simulink model "SF049A_LoaMgr"  (R2013b)
settings: Solver=FixedStepDiscrete  SolverMode=SingleTasking  StartTime=0.0  StopTime=1  FixedStep=0.002  RelTol=1e-3
undefined symbols (not defined in the file): CURRMEASLOAMTGTNMASK_CNT_U08, IVTRLOAMTGTNMASK_CNT_U08, LoaCtrldShtdwn, LoaCurrMeasIdptSigNrFlt, LoaHwTqIdptSigNrFlt, LoaImdtShtdwn, LoaIvtrIdptSigNrFlt, LOAMAXSLEW_ULSPERSEC_F32, LoaMgrCurrIvtrMtgtnRate, LoaMgrCurrIvtrMtgtnSca, LoaMgrCurrIvtrMtgtnScaZeroEna, LoaMgrCurrMeasIdptSig0Resp, LoaMgrCurrMeasIdptSig1Resp, LoaMgrCurrMeasIdptSig2Resp, LoaMgrCurrMeasIdptSigFltThd, LoaMgrCurrMeasMtgtnRate, LoaMgrCurrMeasMtgtnSca, LoaMgrCurrMeasMtgtnScaZeroEna, LoaMgrFadeOutStRate, LoaMgrHwTqIdptSig0NoTqLoaResp, LoaMgrHwTqIdptSig1NoTqLoaResp, LoaMgrHwTqIdptSig2Resp, LoaMgrHwTqIdptSig4Resp, LoaMgrHwTqIdptSigFltThd, LoaMgrHwTqLoaAvlResp, LoaMgrIvtrIdptSig0Resp, LoaMgrIvtrIdptSig1Resp, LoaMgrIvtrIdptSig2Resp, LoaMgrIvtrIdptSigFltThd, LoaMgrIvtrMtgtnRate, LoaMgrIvtrMtgtnSca, LoaMgrIvtrMtgtnScaZeroEna, LoaMgrLimdStRate, LoaMgrLimdStSca, LoaMgrMotAgAvlSnsrlsResp, LoaMgrMotAgIdptSig0NoSnsrlsResp, LoaMgrMotAgIdptSig1NoSnsrlsResp, LoaMgrMotAgIdptSig2Resp, LoaMgrMotAgIdptSig3Resp, LoaMgrMotAgIdptSigFltThd, LoaMgrMotAgMtgtnRate, LoaMgrMotAgMtgtnSca, LoaMgrMotAgMtgtnScaZeroEna, LoaMotAgIdptSigNrFlt, LOASCAONE_ULS_F32, LOASCAZERO_ULS_F32, LoaSt1, LOASTIMDTSHTDWN_CNT_U08, LOASTNORM_CNT_U08, LOASTSWMTGTN_CNT_U08, MAXCURRMEASIDPTSIGALLWD_CNT_U08, MAXHWTQIDPTSIGALLWD_CNT_U08, MAXIVTRIDPTSIGALLWD_CNT_U08, MAXMOTAGMECLIDPTSIGALLWD_CNT_U08, NODEBSTEP_CNT_U16, NtcSts1, SigQlfr1
libraries: simulink x30, NxtrMin x4, NxtrMax x4, NxtrLim x2
(part 6 of 7)

== system SF049A_LoaMgr/LoaMgr/LoaMgrPer1/Assign_Scale/SwMtgtn/OthersTrue ==
  note: Value Assignments
      |   0  neither enabled (shouldn't get here if this is true)
      |   1  MotCurrLoaMtgtnEn
      |   2  IvtrLoaMtgtnEn
      |   3  both enabled
  note: Set case 3 as the default.
  VltgModSrc : Inport  RequirementInfo={} %GIDa_e34c3d9f_9321_4084_85fd_c576df9628c2
  PrevVltgModSrc : Inport  RequirementInfo={} %GIDa_5c8ae546_718f_4248_8614_1d27d062207c  Port=2
  Action Port : ActionPort  ActionType=else
  CopyRight2 : Subsystem  Description=|  mask(Copyright Information){none=on}
      | Copyright info block.                                               
      |                                                                     
      | Place copyright information at the top of every subsystem in design.
      mask prompts: none "No parameters"
      mask help: Place copyright information at the top of every subsystem in design.
      mask Display:
      | NxtrConf = 'Nexteer Confidential';
      | 
      | sys = bdroot; %handle for the current model ("system")
      | first = get_param(sys,'Created');
      | first = first(end-3:end);  %year is last four digits
      | 
      | last = get_param(sys,'LastModifiedDate');
      | if isempty(last)
      |     last = datestr(now,'yyyy');
      | else
      |     last = last(end-3:end);
      | end
      | 
      | if strcmp(first,last)
      |     fprintf('%s -- Copyright %s Nexteer',NxtrConf,first)
      | else
      |     fprintf('%s -- %s%s- %s Nexteer',NxtrConf,char(169),first,last)
      | end
  CurrIvtr : Subsystem  TreatAsAtomicUnit=on
  CurrOnly : Subsystem  TreatAsAtomicUnit=on
  DidItChange : RelationalOperator  RequirementInfo={} %GIDa_9bbcab8f_5ee5_4cef_82f9_f33c7e9d7b46  Operator=~=  OutDataTypeStr=boolean
  IvtrOnly : Subsystem  TreatAsAtomicUnit=on
  RateMerge : Merge  RequirementInfo={} %GIDa_8c2a3104_3c96_4320_aeb7_e788793ea374  Inputs=3
  ScaMerge : Merge  RequirementInfo={} %GIDa_4fe333f2_b27a_4dc4_ad52_ab425be3aec9  Inputs=3
  Switch Case : SwitchCase  RequirementInfo={} %GIDa_a5da75a8_4073_42b0_ad2d_bf75d508884f  CaseConditions={1,2}
  Sca : Outport  RequirementInfo={} %GIDa_8e8336c4_5555_41ff_883b_9885a98480c4
  Rate : Outport  RequirementInfo={} %GIDa_ced75a59_9727_4ef6_b437_f289454741f3  Port=2
  wires:
  ScaMerge/1 -> Sca/1
  RateMerge/1 -> Rate/1
  CurrIvtr/2(Rate) -> RateMerge/3
  IvtrOnly/2(Rate) -> RateMerge/2
  CurrOnly/2(Rate) -> RateMerge/1
  CurrIvtr/1(Sca) -> ScaMerge/3
  IvtrOnly/1(Sca) -> ScaMerge/2
  CurrOnly/1(Sca) -> ScaMerge/1
  Switch Case/3 -> CurrIvtr/Action
  Switch Case/2 -> IvtrOnly/Action
  Switch Case/1 -> CurrOnly/Action
  [Changed] -> CurrIvtr/1(NewValFlg)
  [Changed] -> IvtrOnly/1(NewValFlg)
  [Changed] -> CurrOnly/1(NewValFlg)
  DidItChange/1 -> [Changed]
  PrevVltgModSrc/1 -> DidItChange/2
  VltgModSrc/1 -> DidItChange/1, Switch Case/1

== system SF049A_LoaMgr/LoaMgr/LoaMgrPer1/Calc_Ivtr_State/Ivtr1Sts_ELSE/CopyRight2 ==

== system SF049A_LoaMgr/LoaMgr/LoaMgrPer1/Calc_Ivtr_State/Ivtr1Sts_THEN/CopyRight2 ==

== system SF049A_LoaMgr/LoaMgr/LoaMgrPer1/Calc_Ivtr_State/Ivtr2Sts_ELSE/CopyRight2 ==

== system SF049A_LoaMgr/LoaMgr/LoaMgrPer1/Calc_Ivtr_State/Ivtr2Sts_THEN/CopyRight2 ==

== system SF049A_LoaMgr/LoaMgr/LoaMgrPer1/Latch_Inputs/RngLimCurrMeasIdptSig/Allw ==
  In1 : Inport
  Action Port : ActionPort  ActionType=else
  Out1 : Outport
  wires:
  In1/1 -> Out1/1

== system SF049A_LoaMgr/LoaMgr/LoaMgrPer1/Latch_Inputs/RngLimCurrMeasIdptSig/CopyRight2 ==

== system SF049A_LoaMgr/LoaMgr/LoaMgrPer1/Latch_Inputs/RngLimCurrMeasIdptSig/DftVal ==
  In1 : Inport
  Action Port : ActionPort  ActionType=then
  Out2 : Outport
  wires:
  In1/1 -> Out2/1

== system SF049A_LoaMgr/LoaMgr/LoaMgrPer1/Latch_Inputs/RngLimHwTqIdptSig/Allw ==
  In1 : Inport
  Action Port : ActionPort  ActionType=else
  Out1 : Outport
  wires:
  In1/1 -> Out1/1

== system SF049A_LoaMgr/LoaMgr/LoaMgrPer1/Latch_Inputs/RngLimHwTqIdptSig/CopyRight2 ==

== system SF049A_LoaMgr/LoaMgr/LoaMgrPer1/Latch_Inputs/RngLimHwTqIdptSig/DftVal ==
  In1 : Inport
  Action Port : ActionPort  ActionType=then
  Out2 : Outport
  wires:
  In1/1 -> Out2/1

== system SF049A_LoaMgr/LoaMgr/LoaMgrPer1/Latch_Inputs/RngLimMotAgMecIdptSig/Allw ==
  In1 : Inport
  Action Port : ActionPort  ActionType=else
  Out1 : Outport
  wires:
  In1/1 -> Out1/1

== system SF049A_LoaMgr/LoaMgr/LoaMgrPer1/Latch_Inputs/RngLimMotAgMecIdptSig/CopyRight2 ==

== system SF049A_LoaMgr/LoaMgr/LoaMgrPer1/Latch_Inputs/RngLimMotAgMecIdptSig/DftVal ==
  In1 : Inport
  Action Port : ActionPort  ActionType=then
  Out2 : Outport
  wires:
  In1/1 -> Out2/1

== system SF049A_LoaMgr/LoaMgr/LoaMgrPer1/Request_Responses/CurrMeasResp/CopyRight2 ==

== system SF049A_LoaMgr/LoaMgr/LoaMgrPer1/Request_Responses/CurrMeasResp/Two ==
  Sig2Resp : Inport
  Two : ActionPort  ActionType=case
  CopyRight2 : Subsystem  Description=|  mask(Copyright Information){none=on}
      | Copyright info block.                                               
      |                                                                     
      | Place copyright information at the top of every subsystem in design.
      mask prompts: none "No parameters"
      mask help: Place copyright information at the top of every subsystem in design.
      mask Display:
      | NxtrConf = 'Nexteer Confidential';
      | 
      | sys = bdroot; %handle for the current model ("system")
      | first = get_param(sys,'Created');
      | first = first(end-3:end);  %year is last four digits
      | 
      | last = get_param(sys,'LastModifiedDate');
      | if isempty(last)
      |     last = datestr(now,'yyyy');
      | else
      |     last = last(end-3:end);
      | end
      | 
      | if strcmp(first,last)
      |     fprintf('%s -- Copyright %s Nexteer',NxtrConf,first)
      | else
      |     fprintf('%s -- %s%s- %s Nexteer',NxtrConf,char(169),first,last)
      | end
  CurrMeasResp : Outport
  wires:
  Sig2Resp/1 -> CurrMeasResp/1

== system SF049A_LoaMgr/LoaMgr/LoaMgrPer1/Request_Responses/CurrMeasResp/Zero_or_Invalid ==
  Sig0Resp : Inport
  Default : ActionPort  ActionType=default
  CopyRight2 : Subsystem  Description=|  mask(Copyright Information){none=on}
      | Copyright info block.                                               
      |                                                                     
      | Place copyright information at the top of every subsystem in design.
      mask prompts: none "No parameters"
      mask help: Place copyright information at the top of every subsystem in design.
      mask Display:
      | NxtrConf = 'Nexteer Confidential';
      | 
      | sys = bdroot; %handle for the current model ("system")
      | first = get_param(sys,'Created');
      | first = first(end-3:end);  %year is last four digits
      | 
      | last = get_param(sys,'LastModifiedDate');
      | if isempty(last)
      |     last = datestr(now,'yyyy');
      | else
      |     last = last(end-3:end);
      | end
      | 
      | if strcmp(first,last)
      |     fprintf('%s -- Copyright %s Nexteer',NxtrConf,first)
      | else
      |     fprintf('%s -- %s%s- %s Nexteer',NxtrConf,char(169),first,last)
      | end
  CurrMeasResp : Outport
  wires:
  Sig0Resp/1 -> CurrMeasResp/1

== system SF049A_LoaMgr/LoaMgr/LoaMgrPer1/Request_Responses/CurrMeasResp/one ==
  Sig1Resp : Inport
  one : ActionPort  ActionType=case
  CopyRight2 : Subsystem  Description=|  mask(Copyright Information){none=on}
      | Copyright info block.                                               
      |                                                                     
      | Place copyright information at the top of every subsystem in design.
      mask prompts: none "No parameters"
      mask help: Place copyright information at the top of every subsystem in design.
      mask Display:
      | NxtrConf = 'Nexteer Confidential';
      | 
      | sys = bdroot; %handle for the current model ("system")
      | first = get_param(sys,'Created');
      | first = first(end-3:end);  %year is last four digits
      | 
      | last = get_param(sys,'LastModifiedDate');
      | if isempty(last)
      |     last = datestr(now,'yyyy');
      | else
      |     last = last(end-3:end);
      | end
      | 
      | if strcmp(first,last)
      |     fprintf('%s -- Copyright %s Nexteer',NxtrConf,first)
      | else
      |     fprintf('%s -- %s%s- %s Nexteer',NxtrConf,char(169),first,last)
      | end
  CurrMeasResp : Outport
  wires:
  Sig1Resp/1 -> CurrMeasResp/1

== system SF049A_LoaMgr/LoaMgr/LoaMgrPer1/Request_Responses/HwTqResp/CopyRight2 ==

== system SF049A_LoaMgr/LoaMgr/LoaMgrPer1/Request_Responses/HwTqResp/Four ==
  cal : Inport
  Four : ActionPort  ActionType=case
  CopyRight2 : Subsystem  Description=|  mask(Copyright Information){none=on}
      | Copyright info block.                                               
      |                                                                     
      | Place copyright information at the top of every subsystem in design.
      mask prompts: none "No parameters"
      mask help: Place copyright information at the top of every subsystem in design.
      mask Display:
      | NxtrConf = 'Nexteer Confidential';
      | 
      | sys = bdroot; %handle for the current model ("system")
      | first = get_param(sys,'Created');
      | first = first(end-3:end);  %year is last four digits
      | 
      | last = get_param(sys,'LastModifiedDate');
      | if isempty(last)
      |     last = datestr(now,'yyyy');
      | else
      |     last = last(end-3:end);
      | end
      | 
      | if strcmp(first,last)
      |     fprintf('%s -- Copyright %s Nexteer',NxtrConf,first)
      | else
      |     fprintf('%s -- %s%s- %s Nexteer',NxtrConf,char(169),first,last)
      | end
  HwTqResp : Outport
  wires:
  cal/1 -> HwTqResp/1

== system SF049A_LoaMgr/LoaMgr/LoaMgrPer1/Request_Responses/HwTqResp/Two ==
  cal : Inport
  Two : ActionPort  ActionType=case
  CopyRight2 : Subsystem  Description=|  mask(Copyright Information){none=on}
      | Copyright info block.                                               
      |                                                                     
      | Place copyright information at the top of every subsystem in design.
      mask prompts: none "No parameters"
      mask help: Place copyright information at the top of every subsystem in design.
      mask Display:
      | NxtrConf = 'Nexteer Confidential';
      | 
      | sys = bdroot; %handle for the current model ("system")
      | first = get_param(sys,'Created');
      | first = first(end-3:end);  %year is last four digits
      | 
      | last = get_param(sys,'LastModifiedDate');
      | if isempty(last)
      |     last = datestr(now,'yyyy');
      | else
      |     last = last(end-3:end);
      | end
      | 
      | if strcmp(first,last)
      |     fprintf('%s -- Copyright %s Nexteer',NxtrConf,first)
      | else
      |     fprintf('%s -- %s%s- %s Nexteer',NxtrConf,char(169),first,last)
      | end
  HwTqResp : Outport
  wires:
  cal/1 -> HwTqResp/1

== system SF049A_LoaMgr/LoaMgr/LoaMgrPer1/Request_Responses/HwTqResp/Zero_or_Invalid ==
  TqLoaAvlResp : Inport
  Sig0NoTqLoaResp : Inport  Port=2
  TqLoaAvl : Inport  Port=3
  default : ActionPort  ActionType=default
  " " : Merge  RequirementInfo="{'linktype_rmi_doors' '00012fd5 (/E-STEER Core/SubSystem Specifications/Application Functions - EA4/SF049A Loss of Assist Manager)' '#SF049A_121' 'true' 'REQ:  SF049A_121' '' } %GIDa_5bfa6658_21e2_452d_bd12_27ff54cf6757"
  CopyRight2 : Subsystem  Description=|  mask(Copyright Information){none=on}
      | Copyright info block.                                               
      |                                                                     
      | Place copyright information at the top of every subsystem in design.
      mask prompts: none "No parameters"
      mask help: Place copyright information at the top of every subsystem in design.
      mask Display:
      | NxtrConf = 'Nexteer Confidential';
      | 
      | sys = bdroot; %handle for the current model ("system")
      | first = get_param(sys,'Created');
      | first = first(end-3:end);  %year is last four digits
      | 
      | last = get_param(sys,'LastModifiedDate');
      | if isempty(last)
      |     last = datestr(now,'yyyy');
      | else
      |     last = last(end-3:end);
      | end
      | 
      | if strcmp(first,last)
      |     fprintf('%s -- Copyright %s Nexteer',NxtrConf,first)
      | else
      |     fprintf('%s -- %s%s- %s Nexteer',NxtrConf,char(169),first,last)
      | end
  Ivtr1Inactv_IF : If  RequirementInfo="{'linktype_rmi_doors' '00012fd5 (/E-STEER Core/SubSystem Specifications/Application Functions - EA4/SF049A Loss of Assist Manager)' '#SF049A_121' 'true' 'REQ:  SF049A_121' '' } %GIDa_c6d2db76_b165_49a6_beb7_f28149238192"  IfExpression=u1
  cal1 : Subsystem  RequirementInfo="{'linktype_rmi_doors' '00012fd5 (/E-STEER Core/SubSystem Specifications/Application Functions - EA4/SF049A Loss of Assist Manager)' '#SF049A_121' 'true' 'REQ:  SF049A_121' '' } %GIDa_a20639c0_4bf6_4864_9722_4a86c1b4281d"  TreatAsAtomicUnit=on
      settings: RTWSystemCode=Inline
  cal2 : Subsystem  RequirementInfo="{'linktype_rmi_doors' '00012fd5 (/E-STEER Core/SubSystem Specifications/Application Functions - EA4/SF049A Loss of Assist Manager)' '#SF049A_121' 'true' 'REQ:  SF049A_121' '' } %GIDa_c2c81ba9_b3d8_4db5_b741_5919066dfc70"  TreatAsAtomicUnit=on
      settings: RTWSystemCode=Inline
  HwTqResp : Outport
  wires:
  " "/1 -> HwTqResp/1
  Sig0NoTqLoaResp/1 -> cal2/1(In1)
  TqLoaAvlResp/1 -> cal1/1(In1)
  cal1/1(Out2) -> " "/1
  TqLoaAvl/1 -> Ivtr1Inactv_IF/1
  cal2/1(Out1) -> " "/2
  Ivtr1Inactv_IF/1 -> cal1/Action
  Ivtr1Inactv_IF/2 -> cal2/Action

== system SF049A_LoaMgr/LoaMgr/LoaMgrPer1/Request_Responses/HwTqResp/one ==
  TqLoaAvlResp : Inport
  Sig1NoTqLoaResp : Inport  Port=2
  TqLoaAvl : Inport  Port=3
  one : ActionPort  ActionType=case
  " " : Merge  RequirementInfo={} %GIDa_440ae5c9_fcfa_48ac_8544_293f9d2a3256
  CopyRight2 : Subsystem  Description=|  mask(Copyright Information){none=on}
      | Copyright info block.                                               
      |                                                                     
      | Place copyright information at the top of every subsystem in design.
      mask prompts: none "No parameters"
      mask help: Place copyright information at the top of every subsystem in design.
      mask Display:
      | NxtrConf = 'Nexteer Confidential';
      | 
      | sys = bdroot; %handle for the current model ("system")
      | first = get_param(sys,'Created');
      | first = first(end-3:end);  %year is last four digits
      | 
      | last = get_param(sys,'LastModifiedDate');
      | if isempty(last)
      |     last = datestr(now,'yyyy');
      | else
      |     last = last(end-3:end);
      | end
      | 
      | if strcmp(first,last)
      |     fprintf('%s -- Copyright %s Nexteer',NxtrConf,first)
      | else
      |     fprintf('%s -- %s%s- %s Nexteer',NxtrConf,char(169),first,last)
      | end
  Ivtr1Inactv_IF : If  RequirementInfo={} %GIDa_ab4e5eb2_b673_487c_adb0_5586e49f0879  IfExpression=u1
  cal1 : Subsystem  RequirementInfo={} %GIDa_b5fd7979_0dd1_4a22_9547_ebabb010046f  TreatAsAtomicUnit=on
      settings: RTWSystemCode=Inline
  cal2 : Subsystem  RequirementInfo={} %GIDa_7db3b70f_0bf5_4f15_84c5_d04b7230a7b7  TreatAsAtomicUnit=on
      settings: RTWSystemCode=Inline
  HwTqResp : Outport
  wires:
  " "/1 -> HwTqResp/1
  Sig1NoTqLoaResp/1 -> cal2/1(In1)
  TqLoaAvlResp/1 -> cal1/1(In1)
  cal1/1(Out2) -> " "/1
  TqLoaAvl/1 -> Ivtr1Inactv_IF/1
  cal2/1(Out1) -> " "/2
  Ivtr1Inactv_IF/1 -> cal1/Action
  Ivtr1Inactv_IF/2 -> cal2/Action

== system SF049A_LoaMgr/LoaMgr/LoaMgrPer1/Request_Responses/InvtrResp/CopyRight2 ==

== system SF049A_LoaMgr/LoaMgr/LoaMgrPer1/Request_Responses/InvtrResp/Two ==
  Sig2Resp : Inport
  Two : ActionPort  ActionType=case
  CopyRight2 : Subsystem  Description=|  mask(Copyright Information){none=on}
      | Copyright info block.                                               
      |                                                                     
      | Place copyright information at the top of every subsystem in design.
      mask prompts: none "No parameters"
      mask help: Place copyright information at the top of every subsystem in design.
      mask Display:
      | NxtrConf = 'Nexteer Confidential';
      | 
      | sys = bdroot; %handle for the current model ("system")
      | first = get_param(sys,'Created');
      | first = first(end-3:end);  %year is last four digits
      | 
      | last = get_param(sys,'LastModifiedDate');
      | if isempty(last)
      |     last = datestr(now,'yyyy');
      | else
      |     last = last(end-3:end);
      | end
      | 
      | if strcmp(first,last)
      |     fprintf('%s -- Copyright %s Nexteer',NxtrConf,first)
      | else
      |     fprintf('%s -- %s%s- %s Nexteer',NxtrConf,char(169),first,last)
      | end
  IvtrResp : Outport
  wires:
  Sig2Resp/1 -> IvtrResp/1

== system SF049A_LoaMgr/LoaMgr/LoaMgrPer1/Request_Responses/InvtrResp/Zero_or_Invalid ==
  Sig0Resp : Inport
  Default : ActionPort  ActionType=default
  CopyRight2 : Subsystem  Description=|  mask(Copyright Information){none=on}
      | Copyright info block.                                               
      |                                                                     
      | Place copyright information at the top of every subsystem in design.
      mask prompts: none "No parameters"
      mask help: Place copyright information at the top of every subsystem in design.
      mask Display:
      | NxtrConf = 'Nexteer Confidential';
      | 
      | sys = bdroot; %handle for the current model ("system")
      | first = get_param(sys,'Created');
      | first = first(end-3:end);  %year is last four digits
      | 
      | last = get_param(sys,'LastModifiedDate');
      | if isempty(last)
      |     last = datestr(now,'yyyy');
      | else
      |     last = last(end-3:end);
      | end
      | 
      | if strcmp(first,last)
      |     fprintf('%s -- Copyright %s Nexteer',NxtrConf,first)
      | else
      |     fprintf('%s -- %s%s- %s Nexteer',NxtrConf,char(169),first,last)
      | end
  IvtrResp : Outport
  wires:
  Sig0Resp/1 -> IvtrResp/1

== system SF049A_LoaMgr/LoaMgr/LoaMgrPer1/Request_Responses/InvtrResp/one ==
  Sig1Resp : Inport
  one : ActionPort  ActionType=case
  CopyRight2 : Subsystem  Description=|  mask(Copyright Information){none=on}
      | Copyright info block.                                               
      |                                                                     
      | Place copyright information at the top of every subsystem in design.
      mask prompts: none "No parameters"
      mask help: Place copyright information at the top of every subsystem in design.
      mask Display:
      | NxtrConf = 'Nexteer Confidential';
      | 
      | sys = bdroot; %handle for the current model ("system")
      | first = get_param(sys,'Created');
      | first = first(end-3:end);  %year is last four digits
      | 
      | last = get_param(sys,'LastModifiedDate');
      | if isempty(last)
      |     last = datestr(now,'yyyy');
      | else
      |     last = last(end-3:end);
      | end
      | 
      | if strcmp(first,last)
      |     fprintf('%s -- Copyright %s Nexteer',NxtrConf,first)
      | else
      |     fprintf('%s -- %s%s- %s Nexteer',NxtrConf,char(169),first,last)
      | end
  IvtrResp : Outport
  wires:
  Sig1Resp/1 -> IvtrResp/1

== system SF049A_LoaMgr/LoaMgr/LoaMgrPer1/Request_Responses/MotAgResp/CopyRight2 ==

== system SF049A_LoaMgr/LoaMgr/LoaMgrPer1/Request_Responses/MotAgResp/Three ==
  cal : Inport
  Three : ActionPort  ActionType=case
  CopyRight2 : Subsystem  Description=|  mask(Copyright Information){none=on}
      | Copyright info block.                                               
      |                                                                     
      | Place copyright information at the top of every subsystem in design.
      mask prompts: none "No parameters"
      mask help: Place copyright information at the top of every subsystem in design.
      mask Display:
      | NxtrConf = 'Nexteer Confidential';
      | 
      | sys = bdroot; %handle for the current model ("system")
      | first = get_param(sys,'Created');
      | first = first(end-3:end);  %year is last four digits
      | 
      | last = get_param(sys,'LastModifiedDate');
      | if isempty(last)
      |     last = datestr(now,'yyyy');
      | else
      |     last = last(end-3:end);
      | end
      | 
      | if strcmp(first,last)
      |     fprintf('%s -- Copyright %s Nexteer',NxtrConf,first)
      | else
      |     fprintf('%s -- %s%s- %s Nexteer',NxtrConf,char(169),first,last)
      | end
  MotAgResp : Outport
  wires:
  cal/1 -> MotAgResp/1

== system SF049A_LoaMgr/LoaMgr/LoaMgrPer1/Request_Responses/MotAgResp/Two ==
  cal : Inport
  Two : ActionPort  ActionType=case
  CopyRight2 : Subsystem  Description=|  mask(Copyright Information){none=on}
      | Copyright info block.                                               
      |                                                                     
      | Place copyright information at the top of every subsystem in design.
      mask prompts: none "No parameters"
      mask help: Place copyright information at the top of every subsystem in design.
      mask Display:
      | NxtrConf = 'Nexteer Confidential';
      | 
      | sys = bdroot; %handle for the current model ("system")
      | first = get_param(sys,'Created');
      | first = first(end-3:end);  %year is last four digits
      | 
      | last = get_param(sys,'LastModifiedDate');
      | if isempty(last)
      |     last = datestr(now,'yyyy');
      | else
      |     last = last(end-3:end);
      | end
      | 
      | if strcmp(first,last)
      |     fprintf('%s -- Copyright %s Nexteer',NxtrConf,first)
      | else
      |     fprintf('%s -- %s%s- %s Nexteer',NxtrConf,char(169),first,last)
      | end
  MotAgResp : Outport
  wires:
  cal/1 -> MotAgResp/1

== system SF049A_LoaMgr/LoaMgr/LoaMgrPer1/Request_Responses/MotAgResp/Zero_or_Invalid ==
  MotAgAvlSnsrlsResp : Inport
  MotAgIdptSig0NoResp : Inport  Port=2
  MotAgSnsrlsAvl : Inport  Port=3
  Default : ActionPort  ActionType=default
  " " : Merge  RequirementInfo="{'linktype_rmi_doors' '00012fd5 (/E-STEER Core/SubSystem Specifications/Application Functions - EA4/SF049A Loss of Assist Manager)' '#SF049A_124' 'true' 'REQ:  SF049A_124' '' } %GIDa_f97b5c78_2b89_4252_ada2_558447f79439"
  CopyRight2 : Subsystem  Description=|  mask(Copyright Information){none=on}
      | Copyright info block.                                               
      |                                                                     
      | Place copyright information at the top of every subsystem in design.
      mask prompts: none "No parameters"
      mask help: Place copyright information at the top of every subsystem in design.
      mask Display:
      | NxtrConf = 'Nexteer Confidential';
      | 
      | sys = bdroot; %handle for the current model ("system")
      | first = get_param(sys,'Created');
      | first = first(end-3:end);  %year is last four digits
      | 
      | last = get_param(sys,'LastModifiedDate');
      | if isempty(last)
      |     last = datestr(now,'yyyy');
      | else
      |     last = last(end-3:end);
      | end
      | 
      | if strcmp(first,last)
      |     fprintf('%s -- Copyright %s Nexteer',NxtrConf,first)
      | else
      |     fprintf('%s -- %s%s- %s Nexteer',NxtrConf,char(169),first,last)
      | end
  Ivtr1Inactv_IF : If  RequirementInfo="{'linktype_rmi_doors' '00012fd5 (/E-STEER Core/SubSystem Specifications/Application Functions - EA4/SF049A Loss of Assist Manager)' '#SF049A_124' 'true' 'REQ:  SF049A_124' '' } %GIDa_33e1715d_efda_44a5_a8e3_a1b0953de4a5"  IfExpression=u1
  cal1 : Subsystem  RequirementInfo="{'linktype_rmi_doors' '00012fd5 (/E-STEER Core/SubSystem Specifications/Application Functions - EA4/SF049A Loss of Assist Manager)' '#SF049A_124' 'true' 'REQ:  SF049A_124' '' } %GIDa_6a8a84df_fde8_47d8_b854_0cd4671b0f90"  TreatAsAtomicUnit=on
      settings: RTWSystemCode=Inline
  cal2 : Subsystem  RequirementInfo="{'linktype_rmi_doors' '00012fd5 (/E-STEER Core/SubSystem Specifications/Application Functions - EA4/SF049A Loss of Assist Manager)' '#SF049A_124' 'true' 'REQ:  SF049A_124' '' } %GIDa_ba025aa9_cf38_4a71_985b_5f910ce3ffb4"  TreatAsAtomicUnit=on
      settings: RTWSystemCode=Inline
  MotAgResp : Outport
  wires:
  Ivtr1Inactv_IF/2 -> cal2/Action
  Ivtr1Inactv_IF/1 -> cal1/Action
  cal2/1(Out1) -> " "/2
  MotAgSnsrlsAvl/1 -> Ivtr1Inactv_IF/1
  cal1/1(Out2) -> " "/1
  MotAgAvlSnsrlsResp/1 -> cal1/1(In1)
  MotAgIdptSig0NoResp/1 -> cal2/1(In1)
  " "/1 -> MotAgResp/1

== system SF049A_LoaMgr/LoaMgr/LoaMgrPer1/Request_Responses/MotAgResp/one ==
  MotAgAvlSnsrlsResp : Inport
  MotAgIdptSig1NoResp : Inport  Port=2
  MotAgSnsrlsAvl : Inport  Port=3
  one : ActionPort  ActionType=case
  " " : Merge  RequirementInfo={} %GIDa_26e05d28_98c2_42fa_950d_35dff0512e36
  CopyRight2 : Subsystem  Description=|  mask(Copyright Information){none=on}
      | Copyright info block.                                               
      |                                                                     
      | Place copyright information at the top of every subsystem in design.
      mask prompts: none "No parameters"
      mask help: Place copyright information at the top of every subsystem in design.
      mask Display:
      | NxtrConf = 'Nexteer Confidential';
      | 
      | sys = bdroot; %handle for the current model ("system")
      | first = get_param(sys,'Created');
      | first = first(end-3:end);  %year is last four digits
      | 
      | last = get_param(sys,'LastModifiedDate');
      | if isempty(last)
      |     last = datestr(now,'yyyy');
      | else
      |     last = last(end-3:end);
      | end
      | 
      | if strcmp(first,last)
      |     fprintf('%s -- Copyright %s Nexteer',NxtrConf,first)
      | else
      |     fprintf('%s -- %s%s- %s Nexteer',NxtrConf,char(169),first,last)
      | end
  Ivtr1Inactv_IF : If  RequirementInfo={} %GIDa_e6e2b04c_0731_44c4_b84c_2db766d051ef  IfExpression=u1
  cal1 : Subsystem  RequirementInfo={} %GIDa_d02ffd51_437a_4d1b_823e_9b18f07a7e31  TreatAsAtomicUnit=on
      settings: RTWSystemCode=Inline
  cal2 : Subsystem  RequirementInfo={} %GIDa_53db126b_4fcb_465a_a099_a1de11bfacb7  TreatAsAtomicUnit=on
      settings: RTWSystemCode=Inline
  MotAgResp : Outport
  wires:
  Ivtr1Inactv_IF/2 -> cal2/Action
  Ivtr1Inactv_IF/1 -> cal1/Action
  cal2/1(Out1) -> " "/2
  MotAgSnsrlsAvl/1 -> Ivtr1Inactv_IF/1
  cal1/1(Out2) -> " "/1
  MotAgAvlSnsrlsResp/1 -> cal1/1(In1)
  MotAgIdptSig1NoResp/1 -> cal2/1(In1)
  " "/1 -> MotAgResp/1

== system SF049A_LoaMgr/LoaMgr/LoaMgrPer1/Set_Faults/NTC_Fault1/SetNtcSts ==
  NtcNr : Inport
  NtcStInfo : Inport  Port=2
  NtcSts : Inport  Port=3
  DebStep : Inport  Port=4
  CopyRight2 : Subsystem  Description=|  mask(Copyright Information){none=on}
      | Copyright info block.                                               
      |                                                                     
      | Place copyright information at the top of every subsystem in design.
      mask prompts: none "No parameters"
      mask help: Place copyright information at the top of every subsystem in design.
      mask Display:
      | NxtrConf = 'Nexteer Confidential';
      | 
      | sys = bdroot; %handle for the current model ("system")
      | first = get_param(sys,'Created');
      | first = first(end-3:end);  %year is last four digits
      | 
      | last = get_param(sys,'LastModifiedDate');
      | if isempty(last)
      |     last = datestr(now,'yyyy');
      | else
      |     last = last(end-3:end);
      | end
      | 
      | if strcmp(first,last)
      |     fprintf('%s -- Copyright %s Nexteer',NxtrConf,first)
      | else
      |     fprintf('%s -- %s%s- %s Nexteer',NxtrConf,char(169),first,last)
      | end
  Data Store Write1 : DataStoreWrite  DataStoreName=DebStep
  Data Store Write3 : DataStoreWrite  DataStoreName=Fault1_Status
  Terminator : Terminator
  Terminator1 : Terminator
  wires:
  DebStep/1 -> Data Store Write1/1
  NtcSts/1 -> Data Store Write3/1
  NtcNr/1 -> Terminator/1
  NtcStInfo/1 -> Terminator1/1

== system SF049A_LoaMgr/LoaMgr/LoaMgrPer1/Set_Faults/NTC_Fault2/SetNtcSts ==
  NtcNr : Inport
  NtcStInfo : Inport  Port=2
  NtcSts : Inport  Port=3
  DebStep : Inport  Port=4
  CopyRight2 : Subsystem  Description=|  mask(Copyright Information){none=on}
      | Copyright info block.                                               
      |                                                                     
      | Place copyright information at the top of every subsystem in design.
      mask prompts: none "No parameters"
      mask help: Place copyright information at the top of every subsystem in design.
      mask Display:
      | NxtrConf = 'Nexteer Confidential';
      | 
      | sys = bdroot; %handle for the current model ("system")
      | first = get_param(sys,'Created');
      | first = first(end-3:end);  %year is last four digits
      | 
      | last = get_param(sys,'LastModifiedDate');
      | if isempty(last)
      |     last = datestr(now,'yyyy');
      | else
      |     last = last(end-3:end);
      | end
      | 
      | if strcmp(first,last)
      |     fprintf('%s -- Copyright %s Nexteer',NxtrConf,first)
      | else
      |     fprintf('%s -- %s%s- %s Nexteer',NxtrConf,char(169),first,last)
      | end
  Data Store Write1 : DataStoreWrite  DataStoreName=DebStep
  Data Store Write3 : DataStoreWrite  DataStoreName=Fault2_Status
  Terminator : Terminator
  Terminator1 : Terminator
  wires:
  NtcStInfo/1 -> Terminator1/1
  NtcNr/1 -> Terminator/1
  NtcSts/1 -> Data Store Write3/1
  DebStep/1 -> Data Store Write1/1

== system SF049A_LoaMgr/LoaMgr/LoaMgrPer1/Set_Faults/NTC_Fault3/SetNtcSts ==
  NtcNr : Inport
  NtcStInfo : Inport  Port=2
  NtcSts : Inport  Port=3
  DebStep : Inport  Port=4
  CopyRight2 : Subsystem  Description=|  mask(Copyright Information){none=on}
      | Copyright info block.                                               
      |                                                                     
      | Place copyright information at the top of every subsystem in design.
      mask prompts: none "No parameters"
      mask help: Place copyright information at the top of every subsystem in design.
      mask Display:
      | NxtrConf = 'Nexteer Confidential';
      | 
      | sys = bdroot; %handle for the current model ("system")
      | first = get_param(sys,'Created');
      | first = first(end-3:end);  %year is last four digits
      | 
      | last = get_param(sys,'LastModifiedDate');
      | if isempty(last)
      |     last = datestr(now,'yyyy');
      | else
      |     last = last(end-3:end);
      | end
      | 
      | if strcmp(first,last)
      |     fprintf('%s -- Copyright %s Nexteer',NxtrConf,first)
      | else
      |     fprintf('%s -- %s%s- %s Nexteer',NxtrConf,char(169),first,last)
      | end
  Data Store Write1 : DataStoreWrite  DataStoreName=DebStep
  Data Store Write3 : DataStoreWrite  DataStoreName=Fault3_Status
  Terminator : Terminator
  Terminator1 : Terminator
  wires:
  NtcStInfo/1 -> Terminator1/1
  NtcNr/1 -> Terminator/1
  NtcSts/1 -> Data Store Write3/1
  DebStep/1 -> Data Store Write1/1

== system SF049A_LoaMgr/LoaMgr/LoaMgrPer1/Set_Faults/NTC_Fault4/SetNtcSts ==
  NtcNr : Inport
  NtcStInfo : Inport  Port=2
  NtcSts : Inport  Port=3
  DebStep : Inport  Port=4
  CopyRight2 : Subsystem  Description=|  mask(Copyright Information){none=on}
      | Copyright info block.                                               
      |                                                                     
      | Place copyright information at the top of every subsystem in design.
      mask prompts: none "No parameters"
      mask help: Place copyright information at the top of every subsystem in design.
      mask Display:
      | NxtrConf = 'Nexteer Confidential';
      | 
      | sys = bdroot; %handle for the current model ("system")
      | first = get_param(sys,'Created');
      | first = first(end-3:end);  %year is last four digits
      | 
      | last = get_param(sys,'LastModifiedDate');
      | if isempty(last)
      |     last = datestr(now,'yyyy');
      | else
      |     last = last(end-3:end);
      | end
      | 
      | if strcmp(first,last)
      |     fprintf('%s -- Copyright %s Nexteer',NxtrConf,first)
      | else
      |     fprintf('%s -- %s%s- %s Nexteer',NxtrConf,char(169),first,last)
      | end
  Data Store Write1 : DataStoreWrite  DataStoreName=DebStep
  Data Store Write3 : DataStoreWrite  DataStoreName=Fault4_Status
  Terminator : Terminator
  Terminator1 : Terminator
  wires:
  DebStep/1 -> Data Store Write1/1
  NtcSts/1 -> Data Store Write3/1
  NtcNr/1 -> Terminator/1
  NtcStInfo/1 -> Terminator1/1

== system SF049A_LoaMgr/LoaMgr/LoaMgrPer1/Set_Faults/NTC_Fault5/CopyRight2 ==

== system SF049A_LoaMgr/LoaMgr/LoaMgrPer1/Set_Faults/NTC_Fault6/CopyRight2 ==

== system SF049A_LoaMgr/LoaMgr/LoaMgrPer1/Arbitrate_Responses/CntSwBasdMtgtn/CntMtgtnReq/CopyRight2 ==

== system SF049A_LoaMgr/LoaMgr/LoaMgrPer1/Arbitrate_Responses/CntSwBasdMtgtn/CntMtgtnReq/HwTq_ELSE ==
  In1 : Inport
  Action Port : ActionPort  ActionType=else
  Out1 : Outport
  wires:
  In1/1 -> Out1/1

== system SF049A_LoaMgr/LoaMgr/LoaMgrPer1/Arbitrate_Responses/CntSwBasdMtgtn/CntMtgtnReq/HwTq_THEN ==
  In1 : Inport
  Action Port : ActionPort  ActionType=then
  Out1 : Outport
  wires:
  In1/1 -> Out1/1

== system SF049A_LoaMgr/LoaMgr/LoaMgrPer1/Arbitrate_Responses/CntSwBasdMtgtn/CntMtgtnReq/MotAg_ELSE ==
  In1 : Inport
  Action Port : ActionPort  ActionType=else
  Out1 : Outport
  wires:
  In1/1 -> Out1/1

== system SF049A_LoaMgr/LoaMgr/LoaMgrPer1/Arbitrate_Responses/CntSwBasdMtgtn/CntMtgtnReq/MotAg_THEN ==
  In1 : Inport
  Action Port : ActionPort  ActionType=then
  Out1 : Outport
  wires:
  In1/1 -> Out1/1

== system SF049A_LoaMgr/LoaMgr/LoaMgrPer1/Arbitrate_Responses/CntSwBasdMtgtn/CntMtgtnReq/VltgModReq_ELSE ==
  In1 : Inport
  Action Port : ActionPort  ActionType=else
  Out1 : Outport
  wires:
  In1/1 -> Out1/1

== system SF049A_LoaMgr/LoaMgr/LoaMgrPer1/Arbitrate_Responses/CntSwBasdMtgtn/CntMtgtnReq/VltgModReq_THEN ==
  In1 : Inport
  Action Port : ActionPort  ActionType=then
  Out1 : Outport
  wires:
  In1/1 -> Out1/1

== system SF049A_LoaMgr/LoaMgr/LoaMgrPer1/Arbitrate_Responses/CntSwBasdMtgtn/IllegalCombination/CopyRight2 ==

== system SF049A_LoaMgr/LoaMgr/LoaMgrPer1/Arbitrate_Responses/CntSwBasdMtgtn/OK_to_use/CopyRight2 ==

== system SF049A_LoaMgr/LoaMgr/LoaMgrPer1/Arbitrate_Responses/SelFinalResp/F1/CopyRight2 ==

== system SF049A_LoaMgr/LoaMgr/LoaMgrPer1/Arbitrate_Responses/SelFinalResp/F2/CopyRight2 ==

== system SF049A_LoaMgr/LoaMgr/LoaMgrPer1/Arbitrate_Responses/SelFinalResp/Fade_Out/CopyRight2 ==

== system SF049A_LoaMgr/LoaMgr/LoaMgrPer1/Arbitrate_Responses/SelFinalResp/Norm/CopyRight2 ==

== system SF049A_LoaMgr/LoaMgr/LoaMgrPer1/Arbitrate_Responses/SelFinalResp/Reduced/CopyRight2 ==

== system SF049A_LoaMgr/LoaMgr/LoaMgrPer1/Arbitrate_Responses/SelFinalResp/SwBasd_Mtgtn/CopyRight2 ==

== system SF049A_LoaMgr/LoaMgr/LoaMgrPer1/Assign_Scale/SwMtgtn/HwTqTrue/CopyRight2 ==

== system SF049A_LoaMgr/LoaMgr/LoaMgrPer1/Assign_Scale/SwMtgtn/MaskBooleans/CopyRight2 ==

== system SF049A_LoaMgr/LoaMgr/LoaMgrPer1/Assign_Scale/SwMtgtn/MaskBooleans/CurrMeas_ELSE ==
  In1 : Inport
  Action Port : ActionPort  ActionType=else
  Out1 : Outport
  wires:
  In1/1 -> Out1/1

== system SF049A_LoaMgr/LoaMgr/LoaMgrPer1/Assign_Scale/SwMtgtn/MaskBooleans/CurrMeas_THEN ==
  In1 : Inport
  Action Port : ActionPort  ActionType=then
  Out1 : Outport
  wires:
  In1/1 -> Out1/1

== system SF049A_LoaMgr/LoaMgr/LoaMgrPer1/Assign_Scale/SwMtgtn/MaskBooleans/Ivtr_ELSE ==
  In1 : Inport
  Action Port : ActionPort  ActionType=else
  Out1 : Outport
  wires:
  In1/1 -> Out1/1

== system SF049A_LoaMgr/LoaMgr/LoaMgrPer1/Assign_Scale/SwMtgtn/MaskBooleans/Ivtr_THEN ==
  In1 : Inport
  Action Port : ActionPort  ActionType=then
  Out1 : Outport
  wires:
  In1/1 -> Out1/1

== system SF049A_LoaMgr/LoaMgr/LoaMgrPer1/Assign_Scale/SwMtgtn/MotAgTrue/CopyRight2 ==

== system SF049A_LoaMgr/LoaMgr/LoaMgrPer1/Assign_Scale/SwMtgtn/MotAgTrue/PassThru1 ==
  In1 : Inport
  In2 : Inport  Port=2
  Action Port : ActionPort  ActionType=then
  Sca : Outport
  Rate : Outport  Port=2
  wires:
  In2/1 -> Rate/1
  In1/1 -> Sca/1

== system SF049A_LoaMgr/LoaMgr/LoaMgrPer1/Assign_Scale/SwMtgtn/MotAgTrue/PassThru2 ==
  In1 : Inport
  In2 : Inport  Port=2
  Action Port : ActionPort  ActionType=else
  Sca : Outport
  Rate : Outport  Port=2
  wires:
  In2/1 -> Rate/1
  In1/1 -> Sca/1

== system SF049A_LoaMgr/LoaMgr/LoaMgrPer1/Assign_Scale/SwMtgtn/OthersTrue/CopyRight2 ==

== system SF049A_LoaMgr/LoaMgr/LoaMgrPer1/Assign_Scale/SwMtgtn/OthersTrue/CurrIvtr ==
  NewValFlg : Inport  RequirementInfo={} %GIDa_6dd56434_e9bb_4e70_92c3_53f256375a35
  Action Port : ActionPort  ActionType=default
  Constant1 : Constant  RequirementInfo={} %GIDa_c26ff4c3_9b2d_42cd_8a73_e73906cf7433  Value=LoaMgrCurrIvtrMtgtnRate
  Constant3 : Constant  RequirementInfo={} %GIDa_a49f4269_0df3_42a7_92c8_9ded969204a0  Value=LOASCAZERO_ULS_F32
  Constant4 : Constant  RequirementInfo={} %GIDa_9a4681c8_ac14_4d58_b427_e4fd44fe7aea  Value=LOAMAXSLEW_ULSPERSEC_F32
  Constant5 : Constant  RequirementInfo={} %GIDa_2a4cb365_bee8_412d_80f0_8d3ebb6a1532  Value=LoaMgrCurrIvtrMtgtnScaZeroEna
  Constant6 : Constant  RequirementInfo={} %GIDa_7b8e7c5a_125a_465d_a0d5_a5478ee0ce98  Value=LoaMgrCurrIvtrMtgtnSca
  CopyRight2 : Subsystem  Description=|  mask(Copyright Information){none=on}
      | Copyright info block.                                               
      |                                                                     
      | Place copyright information at the top of every subsystem in design.
      mask prompts: none "No parameters"
      mask help: Place copyright information at the top of every subsystem in design.
      mask Display:
      | NxtrConf = 'Nexteer Confidential';
      | 
      | sys = bdroot; %handle for the current model ("system")
      | first = get_param(sys,'Created');
      | first = first(end-3:end);  %year is last four digits
      | 
      | last = get_param(sys,'LastModifiedDate');
      | if isempty(last)
      |     last = datestr(now,'yyyy');
      | else
      |     last = last(end-3:end);
      | end
      | 
      | if strcmp(first,last)
      |     fprintf('%s -- Copyright %s Nexteer',NxtrConf,first)
      | else
      |     fprintf('%s -- %s%s- %s Nexteer',NxtrConf,char(169),first,last)
      | end
  If : If  RequirementInfo={} %GIDa_324c4790_19e4_441b_b9fa_56dae1a45327  NumInputs=2  IfExpression=u1 & u2
  PassThru1 : Subsystem  RequirementInfo={} %GIDa_6e550954_bcea_4534_b62c_5187013b545f  TreatAsAtomicUnit=on
  PassThru2 : Subsystem  RequirementInfo={} %GIDa_60390cf4_9118_4ada_9140_14c4c310795b  TreatAsAtomicUnit=on
  RateMerge : Merge  RequirementInfo={} %GIDa_a70e2baf_21b0_4515_8500_228af449e03a
  ScaMerge : Merge  RequirementInfo={} %GIDa_a759fa55_284d_4d2c_b257_1dac3a8fda10
  Sca : Outport  RequirementInfo={} %GIDa_41f53cf9_59ce_463b_9636_7eec62d06148
  Rate : Outport  RequirementInfo={} %GIDa_5cbd8a92_4145_4576_883e_d7503e9af478  Port=2
  wires:
  ScaMerge/1 -> Sca/1
  RateMerge/1 -> Rate/1
  NewValFlg/1 -> If/1
  Constant5/1 -> If/2
  Constant3/1 -> PassThru1/1(In1)
  Constant4/1 -> PassThru1/2(In2)
  Constant6/1 -> PassThru2/1(In1)
  Constant1/1 -> PassThru2/2(In2)
  If/1 -> PassThru1/Action
  If/2 -> PassThru2/Action
  PassThru1/1(Sca) -> ScaMerge/1
  PassThru1/2(Rate) -> RateMerge/1
  PassThru2/1(Sca) -> ScaMerge/2
  PassThru2/2(Rate) -> RateMerge/2

== system SF049A_LoaMgr/LoaMgr/LoaMgrPer1/Assign_Scale/SwMtgtn/OthersTrue/CurrOnly ==
  note: IF NewValFlag and Cal are both True THEN
      |      Target scale factor is Zero
      |      Slew rate is instantaneous
      | ELSE
      |      Target scale factor is a cal value
      |      Slew rate is a cal value
      | ENDIF
  note: We could only reach this routine when the combination of s/w-based mitigations changed, making the NewValFlag true.
      | When the flag is true the user may want to drop scale factor instantly to zero and then ramp back up to a target.
  note: If we enter this block on the next loop, the NewValFlag will be FALSE because of the current loop.
      | The user's calibrated scale factor and slew rate will be used.  This means that the slew rate is
      | applied whether the system is slewing down from ONE or up from ZERO.
  NewValFlg : Inport  RequirementInfo={} %GIDa_f087fc8b_f644_4f11_9c46_913b66d21ffd
  Action Port : ActionPort  ActionType=case
  Constant1 : Constant  RequirementInfo={} %GIDa_1030807d_1c0e_4674_afe5_0796a6de07ec  Value=LoaMgrCurrMeasMtgtnRate
  Constant3 : Constant  RequirementInfo={} %GIDa_c5097d7d_98ba_44ea_b9cc_00875abaebba  Value=LOASCAZERO_ULS_F32
  Constant4 : Constant  RequirementInfo={} %GIDa_a936015a_01c2_4556_998c_a6cc28af892b  Value=LOAMAXSLEW_ULSPERSEC_F32
  Constant5 : Constant  RequirementInfo={} %GIDa_aa75c2e3_6275_4f0b_b832_8c37fe5f4582  Value=LoaMgrCurrMeasMtgtnScaZeroEna
  Constant6 : Constant  RequirementInfo={} %GIDa_7722f421_cefc_4daa_a03f_7f61f1b079d1  Value=LoaMgrCurrMeasMtgtnSca
  CopyRight2 : Subsystem  Description=|  mask(Copyright Information){none=on}
      | Copyright info block.                                               
      |                                                                     
      | Place copyright information at the top of every subsystem in design.
      mask prompts: none "No parameters"
      mask help: Place copyright information at the top of every subsystem in design.
      mask Display:
      | NxtrConf = 'Nexteer Confidential';
      | 
      | sys = bdroot; %handle for the current model ("system")
      | first = get_param(sys,'Created');
      | first = first(end-3:end);  %year is last four digits
      | 
      | last = get_param(sys,'LastModifiedDate');
      | if isempty(last)
      |     last = datestr(now,'yyyy');
      | else
      |     last = last(end-3:end);
      | end
      | 
      | if strcmp(first,last)
      |     fprintf('%s -- Copyright %s Nexteer',NxtrConf,first)
      | else
      |     fprintf('%s -- %s%s- %s Nexteer',NxtrConf,char(169),first,last)
      | end
  If : If  RequirementInfo={} %GIDa_4c03382f_3849_4b58_b633_81da7e0dde27  NumInputs=2  IfExpression=u1 & u2
  PassThru1 : Subsystem  RequirementInfo={} %GIDa_fa3df732_5da0_48aa_aa82_01e59d3e20ec  TreatAsAtomicUnit=on
  PassThru2 : Subsystem  RequirementInfo={} %GIDa_c142356f_7e45_4316_a0f3_ce9e567fb8aa  TreatAsAtomicUnit=on
  RateMerge : Merge  RequirementInfo={} %GIDa_76744d5f_6aec_47ec_b8be_546057d11f28
  ScaMerge : Merge  RequirementInfo={} %GIDa_6694feb0_8262_4577_b48a_0840aee5d85c
  Sca : Outport  RequirementInfo={} %GIDa_8fc96b67_933d_40f5_9004_71b54c855907
  Rate : Outport  RequirementInfo={} %GIDa_272833f1_ef92_430d_8660_8113d322bf34  Port=2
  wires:
  ScaMerge/1 -> Sca/1
  RateMerge/1 -> Rate/1
  NewValFlg/1 -> If/1
  Constant5/1 -> If/2
  Constant3/1 -> PassThru1/1(In1)
  Constant4/1 -> PassThru1/2(In2)
  Constant6/1 -> PassThru2/1(In1)
  Constant1/1 -> PassThru2/2(In2)
  If/1 -> PassThru1/Action
  If/2 -> PassThru2/Action
  PassThru1/1(Sca) -> ScaMerge/1
  PassThru1/2(Rate) -> RateMerge/1
  PassThru2/1(Sca) -> ScaMerge/2
  PassThru2/2(Rate) -> RateMerge/2

== system SF049A_LoaMgr/LoaMgr/LoaMgrPer1/Assign_Scale/SwMtgtn/OthersTrue/IvtrOnly ==
  NewValFlg : Inport  RequirementInfo={} %GIDa_3273575a_1857_400c_be36_bf04281c1c03
  Action Port : ActionPort  ActionType=case
  Constant1 : Constant  RequirementInfo={} %GIDa_9f35b5a8_c915_4832_9282_15fc629ce521  Value=LoaMgrIvtrMtgtnRate
  Constant3 : Constant  RequirementInfo={} %GIDa_186fefea_3424_41bc_a139_62b25462ce14  Value=LOASCAZERO_ULS_F32
  Constant4 : Constant  RequirementInfo={} %GIDa_cc1ae4f6_4100_41b6_bafa_b6773fa1f1a7  Value=LOAMAXSLEW_ULSPERSEC_F32
  Constant5 : Constant  RequirementInfo={} %GIDa_584a8d8c_13c8_4476_adf3_baa0387aea5b  Value=LoaMgrIvtrMtgtnScaZeroEna
  Constant6 : Constant  RequirementInfo={} %GIDa_8bf9dc0e_8073_4f58_aa3f_bda34be439cf  Value=LoaMgrIvtrMtgtnSca
  CopyRight2 : Subsystem  Description=|  mask(Copyright Information){none=on}
      | Copyright info block.                                               
      |                                                                     
      | Place copyright information at the top of every subsystem in design.
      mask prompts: none "No parameters"
      mask help: Place copyright information at the top of every subsystem in design.
      mask Display:
      | NxtrConf = 'Nexteer Confidential';
      | 
      | sys = bdroot; %handle for the current model ("system")
      | first = get_param(sys,'Created');
      | first = first(end-3:end);  %year is last four digits
      | 
      | last = get_param(sys,'LastModifiedDate');
      | if isempty(last)
      |     last = datestr(now,'yyyy');
      | else
      |     last = last(end-3:end);
      | end
      | 
      | if strcmp(first,last)
      |     fprintf('%s -- Copyright %s Nexteer',NxtrConf,first)
      | else
      |     fprintf('%s -- %s%s- %s Nexteer',NxtrConf,char(169),first,last)
      | end
  If : If  RequirementInfo={} %GIDa_086c69f3_c4e9_4273_a89c_3799f7b4a971  NumInputs=2  IfExpression=u1 & u2
  PassThru1 : Subsystem  RequirementInfo={} %GIDa_5f621e71_5995_4631_899f_d27afbb99ae7  TreatAsAtomicUnit=on
  PassThru2 : Subsystem  RequirementInfo={} %GIDa_4aff27b5_694f_42ea_9fce_b82b3dc85d0f  TreatAsAtomicUnit=on
  RateMerge : Merge  RequirementInfo={} %GIDa_ab4c95ee_40dc_4b87_87c7_729bebeacbef
  ScaMerge : Merge  RequirementInfo={} %GIDa_50ea305d_078f_472a_9715_32acefd3c0e6
  Sca : Outport  RequirementInfo={} %GIDa_d3e480e5_56fa_46e1_b8d8_0af3cefa4792
  Rate : Outport  RequirementInfo={} %GIDa_084cf5a2_e590_4544_b4d9_7ac842197cd4  Port=2
  wires:
  ScaMerge/1 -> Sca/1
  RateMerge/1 -> Rate/1
  NewValFlg/1 -> If/1
  Constant5/1 -> If/2
  Constant3/1 -> PassThru1/1(In1)
  Constant4/1 -> PassThru1/2(In2)
  Constant6/1 -> PassThru2/1(In1)
  Constant1/1 -> PassThru2/2(In2)
  If/1 -> PassThru1/Action
  If/2 -> PassThru2/Action
  PassThru1/1(Sca) -> ScaMerge/1
  PassThru1/2(Rate) -> RateMerge/1
  PassThru2/1(Sca) -> ScaMerge/2
  PassThru2/2(Rate) -> RateMerge/2

== system SF049A_LoaMgr/LoaMgr/LoaMgrPer1/Request_Responses/CurrMeasResp/Two/CopyRight2 ==

== system SF049A_LoaMgr/LoaMgr/LoaMgrPer1/Request_Responses/CurrMeasResp/Zero_or_Invalid/CopyRight2 ==

== system SF049A_LoaMgr/LoaMgr/LoaMgrPer1/Request_Responses/CurrMeasResp/one/CopyRight2 ==

== system SF049A_LoaMgr/LoaMgr/LoaMgrPer1/Request_Responses/HwTqResp/Four/CopyRight2 ==

== system SF049A_LoaMgr/LoaMgr/LoaMgrPer1/Request_Responses/HwTqResp/Two/CopyRight2 ==

== system SF049A_LoaMgr/LoaMgr/LoaMgrPer1/Request_Responses/HwTqResp/Zero_or_Invalid/CopyRight2 ==
